simulink model "buck_boost_sim"  (R2020a)
settings: Solver=FixedStepAuto  StartTime=0.0  StopTime=sim_duration  FixedStep=1e-3  RelTol=1e-3
undefined symbols (not defined in the file): A, B, C, E, H, k_den, k_num, L, R, sim_duration, ue, x2e
libraries: simulink x2, cstblocks x2
settings Model: Creator=HP  LastModifiedBy=H-BRIDGES

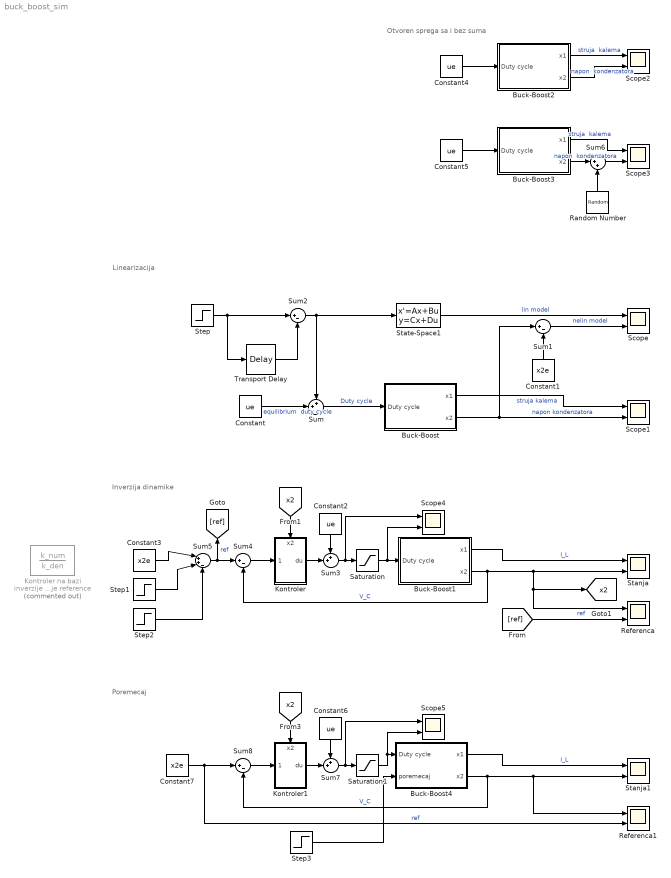
== system buck_boost_sim ==
  note: Otvoren sprega sa i bez suma
  note: Inverzija dinamike
  note: Linearizacija
  note: Poremecaj
  Buck-Boost : Subsystem
  Buck-Boost1 : Subsystem
  Buck-Boost2 : Subsystem
  Buck-Boost3 : Subsystem
  Buck-Boost4 : Subsystem
  Constant{,2,4..6} (5 alike) : Constant  Value=ue
  Constant1 : Constant  Value=x2e
  Constant3 : Constant  Value=x2e
  Constant7 : Constant  Value=x2e
  Kontroler : Subsystem
      settings: PortSchema="{\"entries\":[{\"content\":{\"sides\":[{\"content\":{\"connectorIds\":[\"In1\"]},\"type\":\"ConnectorPlacement.EquallySpacedRectSide\",\"uuid\":\"8063b38c-d7a1-4af9-8550-680c34d00d56\"},{\"content\":{\"connectorIds\":[\"Out1\"],\"side\":\"RIGHT\"},\"type\":\"ConnectorPlacement.EquallySpacedRectSide\",\"uuid\":\"3a9c754f-67ed-4f11-8bdd-a0f7ebf28da2\"},{\"content\":{\"connectorIds\":[\"In2\"],\"side\":\"TOP\"},\"type\":\"ConnectorPlacement.EquallySpacedRectSide\",\"uuid\":\"da304f6d-ed6b-424c-a40d-9baed8f2948f\"}]},\"type\":\"ConnectorPlacement.EquallySpacedConnector\",\"uuid\":\"e076413a-95ae-426a-a24c-afdb174000a4\"}],\"packageUris\":[\"http://schema.mathworks.com/mf0/Connector/19700101\"],\"version\":\"1.0\"}"
  Kontroler na bazi inverzije dinamike za pracenje reference : TransferFcn  Commented=on  Numerator=k_num  Denominator=k_den
  Kontroler1 : Subsystem
      settings: PortSchema="{\"entries\":[{\"content\":{\"sides\":[{\"content\":{\"connectorIds\":[\"In1\"]},\"type\":\"ConnectorPlacement.EquallySpacedRectSide\",\"uuid\":\"8063b38c-d7a1-4af9-8550-680c34d00d56\"},{\"content\":{\"connectorIds\":[\"Out1\"],\"side\":\"RIGHT\"},\"type\":\"ConnectorPlacement.EquallySpacedRectSide\",\"uuid\":\"3a9c754f-67ed-4f11-8bdd-a0f7ebf28da2\"},{\"content\":{\"connectorIds\":[\"In2\"],\"side\":\"TOP\"},\"type\":\"ConnectorPlacement.EquallySpacedRectSide\",\"uuid\":\"da304f6d-ed6b-424c-a40d-9baed8f2948f\"}]},\"type\":\"ConnectorPlacement.EquallySpacedConnector\",\"uuid\":\"e076413a-95ae-426a-a24c-afdb174000a4\"}],\"packageUris\":[\"http://schema.mathworks.com/mf0/Connector/19700101\"],\"version\":\"1.0\"}"
  Random Number : RandomNumber  Variance=(0.05 * abs(x2e))^2  SampleTime=1e-3
  Referenca : Scope  NumInputPorts=2
  Referenca1 : Scope  NumInputPorts=2
  Saturation : Saturate  UpperLimit=1  LowerLimit=0
  Saturation1 : Saturate  UpperLimit=1  LowerLimit=0
  Scope{,1..5} (6 alike) : Scope  NumInputPorts=2
  Stanja : Scope  NumInputPorts=2
  Stanja1 : Scope  NumInputPorts=2
  State-Space1 : StateSpace  A=A  B=B  C=H  D=0  InitialCondition=0
  Step : Step  Time=0.3*sim_duration  After=0.03*ue  SampleTime=0
  Step1 : Step  Time=0.3*sim_duration  After=0.05 * x2e  SampleTime=0
  Step2 : Step  Time=0.4*sim_duration  After=0.1* x2e  SampleTime=0
  Step3 : Step  Time=0.5*sim_duration  After=2*E  SampleTime=0
  Sum : Sum  Inputs=++|
  Sum{1..2,4,8} (4 alike) : Sum  Inputs=|+-
  Sum3 : Sum  Inputs=++|
  Sum5 : Sum  Inputs=|++-
  Sum6 : Sum  Inputs=|++
  Sum7 : Sum  Inputs=++|
  Transport Delay : TransportDelay  DelayTime=0.1*sim_duration  BufferSize=2048
  tag scope: x2=global
  wires:
  Buck-Boost/2(x2) -> Sum1/1, Scope1/2  "napon kondenzatora"
  Sum/1 -> Buck-Boost/1(Duty cycle)  "Duty cycle"
  Constant1/1 -> Sum1/2
  Sum1/1 -> Scope/2  "nelin model"
  State-Space1/1 -> Scope/1  "lin model"
  Constant/1 -> Sum/2  "equilibrium  duty cycle"
  Step/1 -> Transport Delay/1, Sum2/1
  Transport Delay/1 -> Sum2/2
  Sum2/1 -> State-Space1/1, Sum/1
  Buck-Boost/1(x1) -> Scope1/1  "struja kalema"
  Sum3/1 -> Scope4/1, Saturation/1
  Constant2/1 -> Sum3/1
  Buck-Boost1/2(x2) -> [x2], Referenca/1, Stanja/2, Sum4/2  "V_C"
  Buck-Boost1/1(x1) -> Stanja/1  "I_L"
  Constant3/1 -> Sum5/1
  Sum5/1 -> Sum4/1, [ref]  "ref"
  Step1/1 -> Sum5/2
  Step2/1 -> Sum5/3
  Saturation/1 -> Scope4/2, Buck-Boost1/1(Duty cycle)
  Constant4/1 -> Buck-Boost2/1(Duty cycle)
  Buck-Boost3/1(x1) -> Scope3/1  "struja  kalema"
  Constant5/1 -> Buck-Boost3/1(Duty cycle)
  Sum6/1 -> Scope3/2
  Buck-Boost3/2(x2) -> Sum6/1  "napon  kondenzatora"
  Random Number/1 -> Sum6/2
  Buck-Boost2/1(x1) -> Scope2/1  "struja  kalema"
  Buck-Boost2/2(x2) -> Scope2/2  "napon  kondenzatora"
  [ref] -> Referenca/2  "ref"
  Kontroler/1(du) -> Sum3/2
  [x2] -> Kontroler/2(x2)
  Sum4/1 -> Kontroler/1(error)
  [x2] -> Kontroler1/2(x2)
  Kontroler1/1(du) -> Sum7/2
  Buck-Boost4/1(x1) -> Stanja1/1  "I_L"
  Sum8/1 -> Kontroler1/1(error)
  Saturation1/1 -> Scope5/2, Buck-Boost4/1(Duty cycle)
  Constant6/1 -> Sum7/1
  Constant7/1 -> Referenca1/2, Sum8/1  "ref"
  Buck-Boost4/2(x2) -> Referenca1/1, Stanja1/2, Sum8/2  "V_C"
  Sum7/1 -> Scope5/1, Saturation1/1
  Step3/1 -> Buck-Boost4/2(poremecaj)

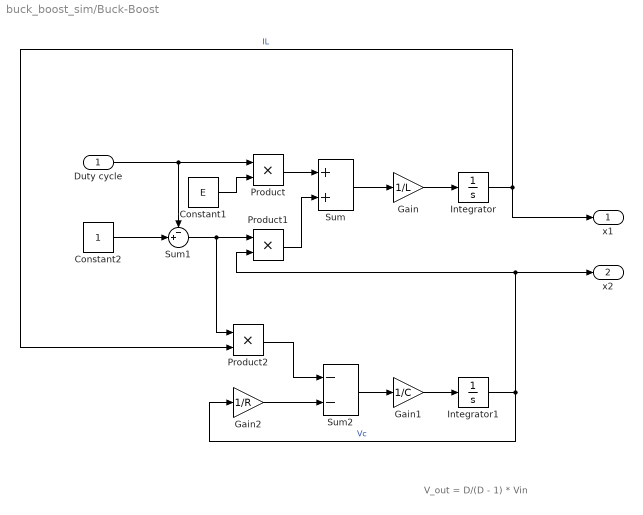
== system buck_boost_sim/Buck-Boost ==
  note: V_out = D/(D - 1) * Vin
  Duty cycle : Inport
  Constant1 : Constant  Value=E
  Constant2 : Constant
  Gain : Gain  Gain=1/L
  Gain1 : Gain  Gain=1/C
  Gain2 : Gain  Gain=1/R
  Integrator : Integrator
  Integrator1 : Integrator
  Product : Product
  Product1 : Product
  Product2 : Product
  Sum : Sum
  Sum1 : Sum  Inputs=-+|
  Sum2 : Sum  Inputs=--
  x1 : Outport
  x2 : Outport  Port=2
  wires:
  Product/1 -> Sum/1
  Product1/1 -> Sum/2
  Sum2/1 -> Gain1/1
  Constant1/1 -> Product/2
  Integrator1/1 -> Gain2/1, x2/1, Product1/2  "Vc"
  Gain1/1 -> Integrator1/1
  Constant2/1 -> Sum1/2
  Integrator/1 -> x1/1, Product2/2  "IL"
  Sum/1 -> Gain/1
  Gain2/1 -> Sum2/2
  Sum1/1 -> Product2/1, Product1/1
  Duty cycle/1 -> Sum1/1, Product/1
  Product2/1 -> Sum2/1
  Gain/1 -> Integrator/1

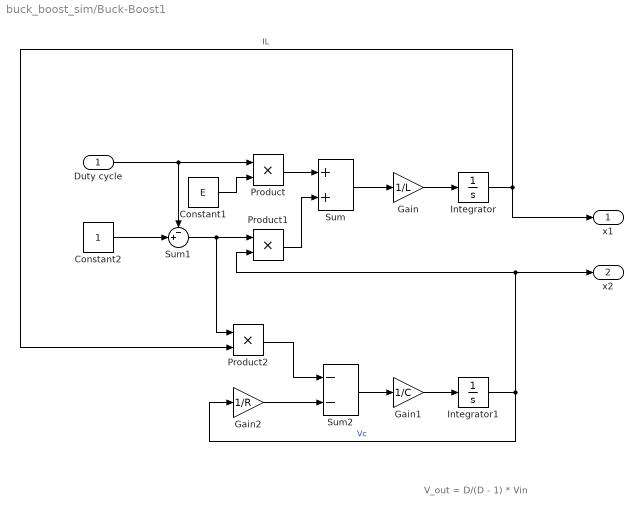
== system buck_boost_sim/Buck-Boost1 ==
  note: V_out = D/(D - 1) * Vin
  Duty cycle : Inport
  Constant1 : Constant  Value=E
  Constant2 : Constant
  Gain : Gain  Gain=1/L
  Gain1 : Gain  Gain=1/C
  Gain2 : Gain  Gain=1/R
  Integrator : Integrator
  Integrator1 : Integrator
  Product : Product
  Product1 : Product
  Product2 : Product
  Sum : Sum
  Sum1 : Sum  Inputs=-+|
  Sum2 : Sum  Inputs=--
  x1 : Outport
  x2 : Outport  Port=2
  wires:
  Product/1 -> Sum/1
  Product1/1 -> Sum/2
  Sum2/1 -> Gain1/1
  Constant1/1 -> Product/2
  Integrator1/1 -> Gain2/1, x2/1, Product1/2  "Vc"
  Gain1/1 -> Integrator1/1
  Constant2/1 -> Sum1/2
  Integrator/1 -> x1/1, Product2/2  "IL"
  Sum/1 -> Gain/1
  Gain2/1 -> Sum2/2
  Sum1/1 -> Product2/1, Product1/1
  Duty cycle/1 -> Sum1/1, Product/1
  Product2/1 -> Sum2/1
  Gain/1 -> Integrator/1

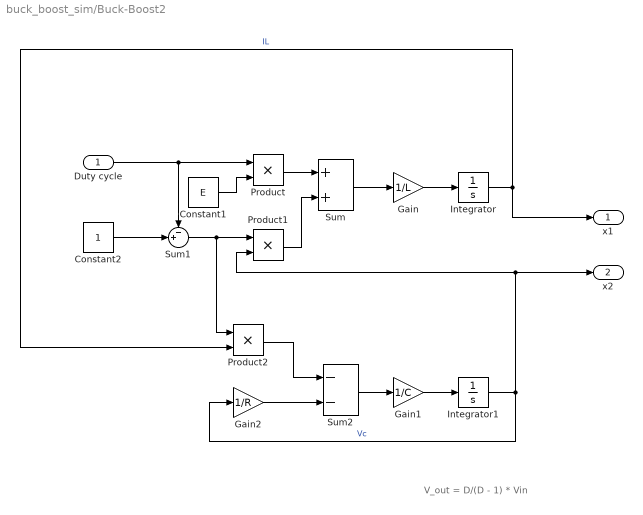
== system buck_boost_sim/Buck-Boost2 ==
  note: V_out = D/(D - 1) * Vin
  Duty cycle : Inport
  Constant1 : Constant  Value=E
  Constant2 : Constant
  Gain : Gain  Gain=1/L
  Gain1 : Gain  Gain=1/C
  Gain2 : Gain  Gain=1/R
  Integrator : Integrator
  Integrator1 : Integrator
  Product : Product
  Product1 : Product
  Product2 : Product
  Sum : Sum
  Sum1 : Sum  Inputs=-+|
  Sum2 : Sum  Inputs=--
  x1 : Outport
  x2 : Outport  Port=2
  wires:
  Product/1 -> Sum/1
  Product1/1 -> Sum/2
  Sum2/1 -> Gain1/1
  Constant1/1 -> Product/2
  Integrator1/1 -> Gain2/1, x2/1, Product1/2  "Vc"
  Gain1/1 -> Integrator1/1
  Constant2/1 -> Sum1/2
  Integrator/1 -> x1/1, Product2/2  "IL"
  Sum/1 -> Gain/1
  Gain2/1 -> Sum2/2
  Sum1/1 -> Product2/1, Product1/1
  Duty cycle/1 -> Sum1/1, Product/1
  Product2/1 -> Sum2/1
  Gain/1 -> Integrator/1

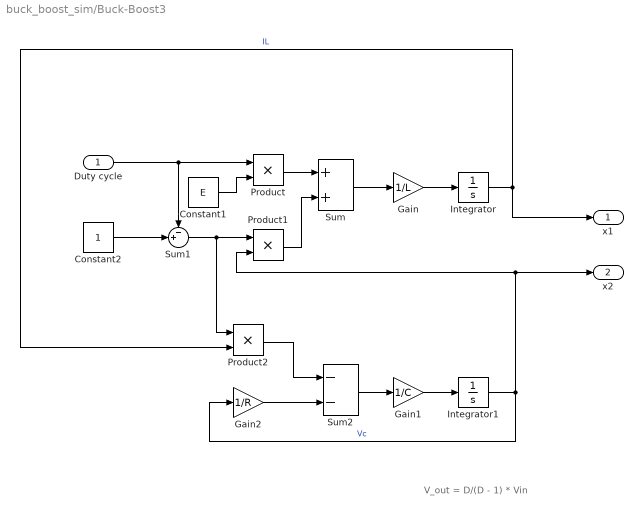
== system buck_boost_sim/Buck-Boost3 ==
  note: V_out = D/(D - 1) * Vin
  Duty cycle : Inport
  Constant1 : Constant  Value=E
  Constant2 : Constant
  Gain : Gain  Gain=1/L
  Gain1 : Gain  Gain=1/C
  Gain2 : Gain  Gain=1/R
  Integrator : Integrator
  Integrator1 : Integrator
  Product : Product
  Product1 : Product
  Product2 : Product
  Sum : Sum
  Sum1 : Sum  Inputs=-+|
  Sum2 : Sum  Inputs=--
  x1 : Outport
  x2 : Outport  Port=2
  wires:
  Product/1 -> Sum/1
  Product1/1 -> Sum/2
  Sum2/1 -> Gain1/1
  Constant1/1 -> Product/2
  Integrator1/1 -> Gain2/1, x2/1, Product1/2  "Vc"
  Gain1/1 -> Integrator1/1
  Constant2/1 -> Sum1/2
  Integrator/1 -> x1/1, Product2/2  "IL"
  Sum/1 -> Gain/1
  Gain2/1 -> Sum2/2
  Sum1/1 -> Product2/1, Product1/1
  Duty cycle/1 -> Sum1/1, Product/1
  Product2/1 -> Sum2/1
  Gain/1 -> Integrator/1

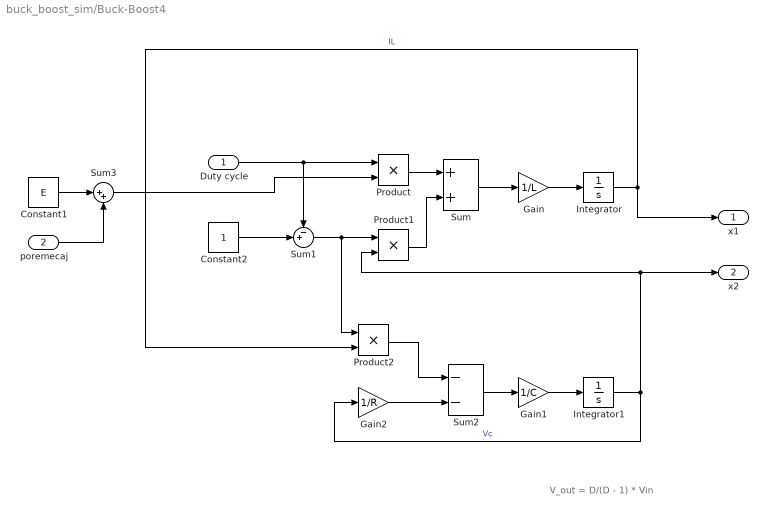
== system buck_boost_sim/Buck-Boost4 ==
  note: V_out = D/(D - 1) * Vin
  Duty cycle : Inport
  poremecaj : Inport  Port=2
  Constant1 : Constant  Value=E
  Constant2 : Constant
  Gain : Gain  Gain=1/L
  Gain1 : Gain  Gain=1/C
  Gain2 : Gain  Gain=1/R
  Integrator : Integrator
  Integrator1 : Integrator
  Product : Product
  Product1 : Product
  Product2 : Product
  Sum : Sum
  Sum1 : Sum  Inputs=-+|
  Sum2 : Sum  Inputs=--
  Sum3 : Sum  Inputs=|++
  x1 : Outport
  x2 : Outport  Port=2
  wires:
  Product/1 -> Sum/1
  Product1/1 -> Sum/2
  Sum2/1 -> Gain1/1
  Integrator1/1 -> Gain2/1, x2/1, Product1/2  "Vc"
  Gain1/1 -> Integrator1/1
  Constant2/1 -> Sum1/2
  Integrator/1 -> x1/1, Product2/2  "IL"
  Sum/1 -> Gain/1
  Gain2/1 -> Sum2/2
  Sum1/1 -> Product2/1, Product1/1
  Duty cycle/1 -> Sum1/1, Product/1
  Product2/1 -> Sum2/1
  Gain/1 -> Integrator/1
  Constant1/1 -> Sum3/1
  Sum3/1 -> Product/2
  poremecaj/1 -> Sum3/2

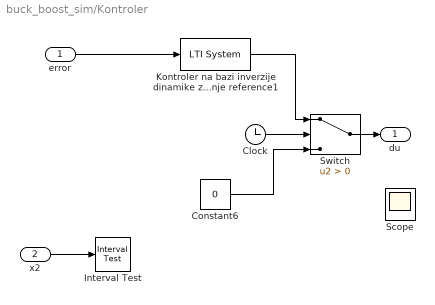
== system buck_boost_sim/Kontroler ==
  error : Inport
  x2 : Inport  Port=2
  Clock : Clock
  Constant6 : Constant  Value=0
  Interval Test : simulink/Logic and Bit Operations/Interval Test  IntervalClosedRight=off  uplimit=0.8*x2e  IntervalClosedLeft=on  lowlimit=-inf  OutDataTypeStr=boolean
  Kontroler na bazi inverzije dinamike za pracenje reference1 : cstblocks/LTI System  sys=K_pracenje_ref  IC=[]
  Scope : Scope
  Switch : Switch  Criteria=u2 > Threshold
  du : Outport
  wires:
  Constant6/1 -> Switch/3
  Kontroler na bazi inverzije dinamike za pracenje reference1/1 -> Switch/1
  error/1 -> Kontroler na bazi inverzije dinamike za pracenje reference1/1
  Switch/1 -> du/1
  x2/1 -> Interval Test/1
  Clock/1 -> Switch/2

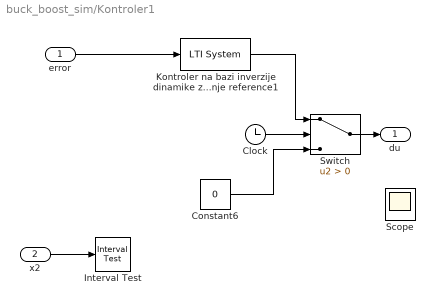
== system buck_boost_sim/Kontroler1 ==
  error : Inport
  x2 : Inport  Port=2
  Clock : Clock
  Constant6 : Constant  Value=0
  Interval Test : simulink/Logic and Bit Operations/Interval Test  IntervalClosedRight=off  uplimit=0.8*x2e  IntervalClosedLeft=on  lowlimit=-inf  OutDataTypeStr=boolean
  Kontroler na bazi inverzije dinamike za pracenje reference1 : cstblocks/LTI System  sys=K_pracenje_ref  IC=[]
  Scope : Scope
  Switch : Switch  Criteria=u2 > Threshold
  du : Outport
  wires:
  Constant6/1 -> Switch/3
  Kontroler na bazi inverzije dinamike za pracenje reference1/1 -> Switch/1
  error/1 -> Kontroler na bazi inverzije dinamike za pracenje reference1/1
  Switch/1 -> du/1
  x2/1 -> Interval Test/1
  Clock/1 -> Switch/2
